simulink model "generic_uservehicle_truck"  (Simulink 10.3)
settings: Solver=ode45  StartTime=0.0  StopTime=inf  RelTol=1e-3  EnableMultiTasking=on
(part 1 of 4)
settings Model: Creator=fh  ModifiedByFormat=IPG  LastModifiedBy=IPG  MultithreadedSim=on  ExtModeAutoUpdateStatusClock=off
settings DataIOCC: LimitDataPoints=on  SignalLoggingName=sigsOut
settings OptimizationCC: BooleanDataType=off  InitFltsAndDblsToZero=on
settings DebuggingCC: SaveWithParameterizedLinksMsg=none  SignalResolutionControl=TryResolveAllWithWarning  MultiTaskDSMMsg=warning  MultiTaskCondExecSysMsg=none  SFExecutionAtInitializationDiag=warning
settings HardwareCC: TargetUnknown=on
settings CodeAppCC: MaxIdLength=63
settings GRTTargetCC: TargetFcnLib=ansi_tfl_tmw.mat

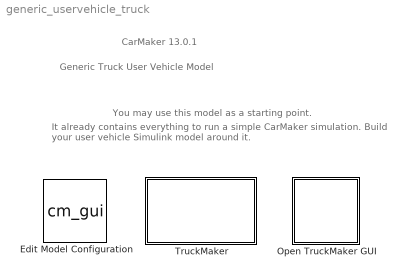
== system generic_uservehicle_truck ==
  note: Generic Truck User Vehicle Model
  note: CarMaker 13.0.1
  note: You may use this model as a starting point.
  note: It already contains everything to run a simple CarMaker simulation.
      | Build your user vehicle Simulink model around it.
  Edit Model Configuration : S-Function  FunctionName=cm_gui  SFunctionDeploymentMode=off  EnableBusSupport=off
      settings: OpenFcn=cmmodelconf('edit');
      mask Display: image(imread('ModelConfig.png'));
  Open TruckMaker GUI : Subsystem  LoadFcn=if ~length(which('cmself')), cmenv; end
      settings: OpenFcn=cmblockmagic('gui_fix_display'); TM_Simulink
      mask Display: image(imread('TruckMakerGUI.png'));
  TruckMaker : Subsystem  TreatAsAtomicUnit=on
      mask Display: image(imread('TruckMakerSys.png'));

== system generic_uservehicle_truck/Open TruckMaker GUI ==
  S-Function : S-Function  FunctionName=cm_gui  SFunctionDeploymentMode=off  EnableBusSupport=off

== system generic_uservehicle_truck/TruckMaker ==
  CM_FIRST : Subsystem
  CM_LAST : Subsystem
  DrivMan : Subsystem
  Ground : Ground
  Terminator : Terminator
  Vehicle : Subsystem
  VehicleControl : Subsystem
  wires:
  DrivMan/2(DrivMan.Out) -> VehicleControl/2(DrivMan.In)
  DrivMan/1(Sync_Out) -> VehicleControl/1(Sync_In)
  CM_FIRST/2(Env.Misc) -> DrivMan/2(Env.Misc)
  CM_FIRST/1(Sync_Out) -> DrivMan/1(Sync_In)
  CM_LAST/1(Sync_Out) -> Terminator/1
  Ground/1 -> CM_FIRST/1(Sync_In)
  Vehicle/1(Sync_Out) -> CM_LAST/1(Sync_In)
  VehicleControl/1(Sync_Out) -> Vehicle/1(Sync_In)
  VehicleControl/3(VhclCtrl.Steering) -> Vehicle/3(VhclCtrl.Steering)
  VehicleControl/4(Vhcl.Wheel.In) -> Vehicle/4(Vhcl.Wheel.In)
  VehicleControl/5(Vhcl.Misc) -> Vehicle/5(Vhcl.Misc)
  VehicleControl/6(VhclCtrl.Brake) -> Vehicle/6(VhclCtrl.Brake)
  VehicleControl/7(VhclCtrl.PT) -> Vehicle/7(VhclCtrl.PT)
  VehicleControl/2(Vhcl.Model.Source) -> Vehicle/2(Vhcl.Model.Source)

== system generic_uservehicle_truck/TruckMaker/CM_FIRST ==
  Sync_In : Inport
  BusCreator1 : BusCreator  Inputs=8
  BusCreator2 : BusCreator  Inputs=6
  Demux1 : Demux  Outputs=14
      settings: DisplayOption=none
  Environment : S-Function  FunctionName=TM_Sfun  Parameters='Environment'  SFunctionDeploymentMode=off  EnableBusSupport=off
  IoIn : S-Function  FunctionName=TM_Sfun  Parameters='IoIn'  SFunctionDeploymentMode=off  EnableBusSupport=off
  Terminator : Terminator
  Sync_Out : Outport  VectorParamsAs1DForOutWhenUnconnected=off
  Env.Misc : Outport  Port=2  VectorParamsAs1DForOutWhenUnconnected=off
  wires:
  BusCreator2/1 -> Terminator/1  "IF Environment (in)"
  BusCreator1/1 -> Env.Misc/1
  Demux1/14 -> BusCreator2/6  "Env sRoad"
  Demux1/13 -> BusCreator2/5  "Env PoI_GCS Elev"
  Demux1/12 -> BusCreator2/4  "Env PoI_GCS Lat"
  Demux1/11 -> BusCreator2/3  "Env PoI_GCS Long"
  Demux1/10 -> BusCreator2/2  "Env Time"
  Demux1/9 -> BusCreator2/1  "Env yDay"
  Demux1/8 -> BusCreator1/8  "Env WindVel_tot z"
  Demux1/7 -> BusCreator1/7  "Env WindVel_tot y"
  Demux1/6 -> BusCreator1/6  "Env WindVel_tot x"
  Demux1/5 -> BusCreator1/5  "Env SolarRadiation"
  Demux1/4 -> BusCreator1/4  "Env AirHumidity"
  Demux1/3 -> BusCreator1/3  "Env AirPressure"
  Demux1/2 -> BusCreator1/2  "Env AirDensity"
  Demux1/1 -> BusCreator1/1  "Env Temperature"
  Environment/2 -> Demux1/1
  Environment/1 -> Sync_Out/1
  IoIn/1 -> Environment/1
  Sync_In/1 -> IoIn/1

== system generic_uservehicle_truck/TruckMaker/CM_LAST ==
  Sync_In : Inport
  CM_User : S-Function  FunctionName=TM_Sfun  Parameters='CM_User'  SFunctionDeploymentMode=off  EnableBusSupport=off
  IoOut : S-Function  FunctionName=TM_Sfun  Parameters='IoOut'  SFunctionDeploymentMode=off  EnableBusSupport=off
  Sync_Out : Outport  VectorParamsAs1DForOutWhenUnconnected=off
  wires:
  IoOut/1 -> Sync_Out/1
  CM_User/1 -> IoOut/1
  Sync_In/1 -> CM_User/1

== system generic_uservehicle_truck/TruckMaker/DrivMan ==
  note: There's rarely a reason to override DrivMan signals.
      | Use the VehicleControl interface for this purpose.
  Sync_In : Inport
  Env.Misc : Inport  Port=2
  BusCreator : BusCreator  Inputs=20
  Demux : Demux  Outputs=20
      settings: DisplayOption=none
  DrivMan : S-Function  FunctionName=TM_Sfun  Parameters='DrivMan'  SFunctionDeploymentMode=off  EnableBusSupport=off
  Sync_Out : Outport  VectorParamsAs1DForOutWhenUnconnected=off
  DrivMan.Out : Outport  Port=2  VectorParamsAs1DForOutWhenUnconnected=off
  wires:
  Demux/8 -> BusCreator/8  "DrivMan SelectorCtrl"
  Demux/7 -> BusCreator/7  "DrivMan UserSignal4"
  Demux/6 -> BusCreator/6  "DrivMan UserSignal3"
  Demux/5 -> BusCreator/5  "DrivMan UserSignal2"
  Demux/4 -> BusCreator/4  "DrivMan UserSignal1"
  Demux/3 -> BusCreator/3  "DrivMan UserSignal0"
  Demux/2 -> BusCreator/2  "DrivMan Key"
  Demux/1 -> BusCreator/1  "DrivMan SST"
  Env.Misc/1 -> DrivMan/2
  Sync_In/1 -> DrivMan/1
  DrivMan/1 -> Sync_Out/1
  BusCreator/1 -> DrivMan.Out/1
  DrivMan/2 -> Demux/1
  Demux/9 -> BusCreator/9  "DrivMan DigitalSelectorCtrl0"
  Demux/10 -> BusCreator/10  "DrivMan DigitalSelectorCtrl1"
  Demux/11 -> BusCreator/11  "DrivMan DigitalSelectorCtrl2"
  Demux/20 -> BusCreator/20  "DrivMan Steering Trq"
  Demux/19 -> BusCreator/19  "DrivMan Steering AngAcc"
  Demux/18 -> BusCreator/18  "DrivMan Steering AngVel"
  Demux/17 -> BusCreator/17  "DrivMan Steering Ang"
  Demux/16 -> BusCreator/16  "DrivMan Gas"
  Demux/15 -> BusCreator/15  "DrivMan Clutch"
  Demux/14 -> BusCreator/14  "DrivMan BrakePark"
  Demux/13 -> BusCreator/13  "DrivMan Brake"
  Demux/12 -> BusCreator/12  "DrivMan GearNo"

== system generic_uservehicle_truck/TruckMaker/Vehicle ==
  note: The enabled subsystems allow for simultaneous availability of more than one vehicle.
      | Which one to use will be determined by the vehicle data set of the Test Run.
      | If this functionality is not needed, you may simplify your model by using
      | the relevant subsystem of the three as a drop-in replacement for the
      | 'Vehicle' subsystem you're currently looking at, as is done in most of the
      | CarMaker for Simulink example models.
      |
      | PLEASE NOTE: In CarMaker HIL-ds100x vehicle switching depending on
      | the vehicle data set is not available. To run the user vehicle, the command
      | line option -disablevehicle in the Model Configuration block is required.
  Sync_In : Inport
  Vhcl.Model.Source : Inport  Port=2
  VhclCtrl.Steering : Inport  Port=3
  Vhcl.Wheel.In : Inport  Port=4
  Vhcl.Misc : Inport  Port=5
  VhclCtrl.Brake : Inport  Port=6
  VhclCtrl.PT : Inport  Port=7
  IPG Vehicle : Subsystem
  Multiport Switch : MultiPortSwitch  InputSameDT=on
  User Vehicle (CM4SL) : Subsystem  TreatAsAtomicUnit=on
  User Vehicle (ModelMgr) : Subsystem  TreatAsAtomicUnit=on
  VehicleSource_BuiltIn : Subsystem  mask(Compare To Constant){relop===, const=1, OutDataTypeStr=boolean, ZeroCross=off}
      mask prompts: relop "Simulink:masks:Operator_MP"; const "Simulink:masks:ConstantValue_MP"; OutDataTypeStr "Simulink:masks:OutputDataType_MP"; ZeroCross "Simulink:masks:EnableZerocrossingDetection_MP"
      mask help: Simulink:masks:CompareToConstant_MD
      mask init:
      | blkName = gcb;
      | 
      | if strcmp(get_param(gcbh,'OutDataTypeStr'),'boolean')
      | 	setValue = 'boolean';
      | else
      | 	setValue = 'fixdt(0, 8)';
      | end
      | 
      | set_param([blkName,'/Compare'],'relop',relop, ...
      | 	'OutDataTypeStr', setValue, 'ZeroCross', ZeroCross);
      | 
      | str = [relop,' C']; %default
      | 
      | const_str = get_param(blkName, 'const');
      | 
      | if isempty(strfind(const_str, ' ')) && isempty(strfind(const_str, ','))
      |     % scalar or single expression
      |     if isempty(str2num(const_str))
      |         %expression
      |         str = [relop, ' ', const_str];
      |     elseif length(const) == 1
      |         str = [relop,' ',num2str(double(const))];
      |     end
      | end
      mask TypeOptions relop: == | ~= | < | <= | >= | >
      mask TypeOptions OutDataTypeStr: Simulink:masks:uint8 | Simulink:masks:boolean
      mask Callback ZeroCross: sl('zeroCrossEnable', gcbh);
      mask Display: disp(str)
  VehicleSource_CM4SL : Subsystem  mask(Compare To Constant){relop===, const=3, OutDataTypeStr=boolean, ZeroCross=off}
      mask prompts: relop "Simulink:masks:Operator_MP"; const "Simulink:masks:ConstantValue_MP"; OutDataTypeStr "Simulink:masks:OutputDataType_MP"; ZeroCross "Simulink:masks:EnableZerocrossingDetection_MP"
      mask help: Simulink:masks:CompareToConstant_MD
      mask init: same as generic_uservehicle_truck/TruckMaker/Vehicle/VehicleSource_BuiltIn
      mask TypeOptions relop: == | ~= | < | <= | >= | >
      mask TypeOptions OutDataTypeStr: Simulink:masks:uint8 | Simulink:masks:boolean
      mask Callback ZeroCross: sl('zeroCrossEnable', gcbh);
      mask Display: disp(str)
  VehicleSource_ModelMgr : Subsystem  mask(Compare To Constant){relop===, const=2, OutDataTypeStr=boolean, ZeroCross=off}
      mask prompts: relop "Simulink:masks:Operator_MP"; const "Simulink:masks:ConstantValue_MP"; OutDataTypeStr "Simulink:masks:OutputDataType_MP"; ZeroCross "Simulink:masks:EnableZerocrossingDetection_MP"
      mask help: Simulink:masks:CompareToConstant_MD
      mask init: same as generic_uservehicle_truck/TruckMaker/Vehicle/VehicleSource_BuiltIn
      mask TypeOptions relop: == | ~= | < | <= | >= | >
      mask TypeOptions OutDataTypeStr: Simulink:masks:uint8 | Simulink:masks:boolean
      mask Callback ZeroCross: sl('zeroCrossEnable', gcbh);
      mask Display: disp(str)
  Sync_Out : Outport  VectorParamsAs1DForOutWhenUnconnected=off
  wires:
  VhclCtrl.Steering/1 -> User Vehicle (CM4SL)/3(VhclCtrl.Steering), User Vehicle (ModelMgr)/3(VhclCtrl.Steering), IPG Vehicle/3(VhclCtrl.Steering)
  Vhcl.Wheel.In/1 -> User Vehicle (CM4SL)/4(Vhcl.Wheel.In), User Vehicle (ModelMgr)/4(Vhcl.Wheel.In), IPG Vehicle/4(Vhcl.Wheel.In)
  Vhcl.Misc/1 -> User Vehicle (CM4SL)/5(Vhcl.Misc), User Vehicle (ModelMgr)/5(Vhcl.Misc), IPG Vehicle/5(Vhcl.Misc)
  VehicleSource_BuiltIn/1(y) -> IPG Vehicle/Enable
  VhclCtrl.Brake/1 -> User Vehicle (CM4SL)/6(VhclCtrl.Brake), User Vehicle (ModelMgr)/6(VhclCtrl.Brake), IPG Vehicle/6(VhclCtrl.Brake)
  VhclCtrl.PT/1 -> User Vehicle (CM4SL)/7(VhclCtrl.PT), User Vehicle (ModelMgr)/7(VhclCtrl.PT), IPG Vehicle/7(VhclCtrl.PT)
  Sync_In/1 -> User Vehicle (CM4SL)/1(Sync_In), User Vehicle (ModelMgr)/1(Sync_In), IPG Vehicle/1(Sync_In)
  Vhcl.Model.Source/1 -> User Vehicle (CM4SL)/2(Vhcl.Model.Source), VehicleSource_ModelMgr/1(u), VehicleSource_BuiltIn/1(u), Multiport Switch/1, IPG Vehicle/2(Vhcl.Model.Source), User Vehicle (ModelMgr)/2(Vhcl.Model.Source), VehicleSource_CM4SL/1(u)
  VehicleSource_CM4SL/1(y) -> User Vehicle (CM4SL)/Enable
  VehicleSource_ModelMgr/1(y) -> User Vehicle (ModelMgr)/Enable
  IPG Vehicle/1(Sync_Out) -> Multiport Switch/2
  User Vehicle (ModelMgr)/1(Sync_Out) -> Multiport Switch/3
  User Vehicle (CM4SL)/1(Sync_Out) -> Multiport Switch/4
  Multiport Switch/1 -> Sync_Out/1

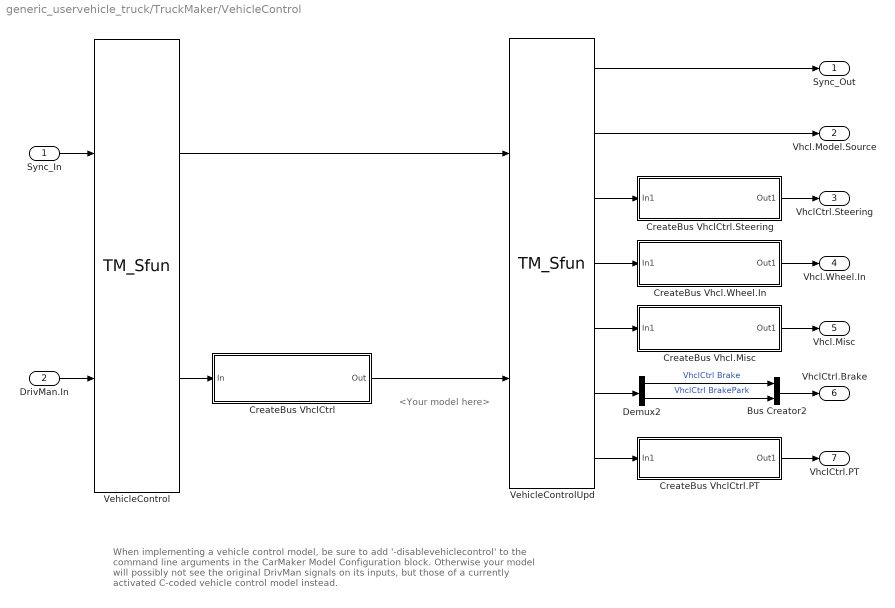
== system generic_uservehicle_truck/TruckMaker/VehicleControl ==
  note: <Your model here>
  note: When implementing a vehicle control model,
      | be sure to add '-disablevehiclecontrol' to the command line arguments
      | in the CarMaker Model Configuration block.
      | Otherwise your model will possibly not see the original DrivMan signals
      | on its inputs, but those of a currently activated C-coded vehicle control model instead.
  Sync_In : Inport
  DrivMan.In : Inport  Port=2
  Bus Creator2 : BusCreator  Inputs=2
  CreateBus Vhcl.Misc : Subsystem
  CreateBus Vhcl.Wheel.In : Subsystem
  CreateBus VhclCtrl : Subsystem
  CreateBus VhclCtrl.PT : Subsystem
  CreateBus VhclCtrl.Steering : Subsystem
  Demux2 : Demux  Outputs=2
      settings: DisplayOption=none
  VehicleControl : S-Function  FunctionName=TM_Sfun  Parameters='VehicleControl'  SFunctionDeploymentMode=off  EnableBusSupport=off
  VehicleControlUpd : S-Function  FunctionName=TM_Sfun  Parameters='VehicleControlUpd'  SFunctionDeploymentMode=off  EnableBusSupport=off
  Sync_Out : Outport  VectorParamsAs1DForOutWhenUnconnected=off
  Vhcl.Model.Source : Outport  Port=2  VectorParamsAs1DForOutWhenUnconnected=off
  VhclCtrl.Steering : Outport  Port=3  VectorParamsAs1DForOutWhenUnconnected=off
  Vhcl.Wheel.In : Outport  Port=4  VectorParamsAs1DForOutWhenUnconnected=off
  Vhcl.Misc : Outport  Port=5  VectorParamsAs1DForOutWhenUnconnected=off
  VhclCtrl.Brake : Outport  Port=6  VectorParamsAs1DForOutWhenUnconnected=off
  VhclCtrl.PT : Outport  Port=7  VectorParamsAs1DForOutWhenUnconnected=off
  wires:
  VehicleControlUpd/2 -> Vhcl.Model.Source/1
  VehicleControlUpd/4 -> CreateBus Vhcl.Wheel.In/1(In1)
  VehicleControlUpd/5 -> CreateBus Vhcl.Misc/1(In1)
  VehicleControlUpd/6 -> Demux2/1
  VehicleControlUpd/7 -> CreateBus VhclCtrl.PT/1(In1)
  VehicleControlUpd/3 -> CreateBus VhclCtrl.Steering/1(In1)
  CreateBus Vhcl.Misc/1(Out1) -> Vhcl.Misc/1
  CreateBus Vhcl.Wheel.In/1(Out1) -> Vhcl.Wheel.In/1
  DrivMan.In/1 -> VehicleControl/2
  CreateBus VhclCtrl/1(Out) -> VehicleControlUpd/2
  VehicleControl/1 -> VehicleControlUpd/1
  VehicleControl/2 -> CreateBus VhclCtrl/1(In)
  Sync_In/1 -> VehicleControl/1
  CreateBus VhclCtrl.PT/1(Out1) -> VhclCtrl.PT/1
  Bus Creator2/1 -> VhclCtrl.Brake/1
  CreateBus VhclCtrl.Steering/1(Out1) -> VhclCtrl.Steering/1
  VehicleControlUpd/1 -> Sync_Out/1
  Demux2/2 -> Bus Creator2/2  "VhclCtrl BrakePark"
  Demux2/1 -> Bus Creator2/1  "VhclCtrl Brake"

== system generic_uservehicle_truck/TruckMaker/Vehicle/IPG Vehicle ==
  Sync_In : Inport
  Vhcl.Model.Source : Inport  Port=2
  VhclCtrl.Steering : Inport  Port=3
  Vhcl.Wheel.In : Inport  Port=4
  Vhcl.Misc : Inport  Port=5
  VhclCtrl.Brake : Inport  Port=6
  VhclCtrl.PT : Inport  Port=7
  Enable : EnablePort
  Brake : Subsystem
  CarAndTrailer : Subsystem
  PowerTrain : Subsystem
  Stop Simulation : Stop
  VehicleSource_BuiltIn : Subsystem  mask(Compare To Constant){relop=~=, const=1, OutDataTypeStr=boolean, ZeroCross=off}
      mask prompts: relop "Simulink:masks:Operator_MP"; const "Simulink:masks:ConstantValue_MP"; OutDataTypeStr "Simulink:masks:OutputDataType_MP"; ZeroCross "Simulink:masks:EnableZerocrossingDetection_MP"
      mask help: Simulink:masks:CompareToConstant_MD
      mask init: same as generic_uservehicle_truck/TruckMaker/Vehicle/VehicleSource_BuiltIn
      mask TypeOptions relop: == | ~= | < | <= | >= | >
      mask TypeOptions OutDataTypeStr: Simulink:masks:uint8 | Simulink:masks:boolean
      mask Callback ZeroCross: sl('zeroCrossEnable', gcbh);
      mask Display: disp(str)
  Sync_Out : Outport  VectorParamsAs1DForOutWhenUnconnected=off
  wires:
  VhclCtrl.PT/1 -> PowerTrain/3(VhclCtrl.PT)
  Brake/1(Sync_Out) -> PowerTrain/1(Sync_In)
  CarAndTrailer/1(Sync_Out) -> Brake/1(Sync_In)
  CarAndTrailer/2(Brake.IF.In) -> Brake/2(Brake.IF.In)
  VhclCtrl.Brake/1 -> Brake/3(VhclCtrl.Brake)
  PowerTrain/1(Sync_Out) -> Sync_Out/1
  Vhcl.Misc/1 -> CarAndTrailer/4(Vhcl.Misc)
  Vhcl.Wheel.In/1 -> CarAndTrailer/3(Vhcl.Wheel.In)
  VhclCtrl.Steering/1 -> CarAndTrailer/2(VhclCtrl.Steering)
  Sync_In/1 -> CarAndTrailer/1(Sync_In)
  Vhcl.Model.Source/1 -> VehicleSource_BuiltIn/1(u)
  VehicleSource_BuiltIn/1(y) -> Stop Simulation/1
  Brake/2(Vhcl.Wheel.PT) -> PowerTrain/2(Vhcl.Wheel.PT)

== system generic_uservehicle_truck/TruckMaker/Vehicle/User Vehicle (CM4SL) ==
  Sync_In : Inport
  Vhcl.Model.Source : Inport  Port=2
  VhclCtrl.Steering : Inport  Port=3
  Vhcl.Wheel.In : Inport  Port=4
  Vhcl.Misc : Inport  Port=5
  VhclCtrl.Brake : Inport  Port=6
  VhclCtrl.PT : Inport  Port=7
  Enable : EnablePort
  Brake : Subsystem
  CarAndTrailer : Subsystem
  PowerTrain : Subsystem
  Stop Simulation : Stop
  VehicleSource_CM4SL : Subsystem  mask(Compare To Constant){relop=~=, const=3, OutDataTypeStr=boolean, ZeroCross=off}
      mask prompts: relop "Simulink:masks:Operator_MP"; const "Simulink:masks:ConstantValue_MP"; OutDataTypeStr "Simulink:masks:OutputDataType_MP"; ZeroCross "Simulink:masks:EnableZerocrossingDetection_MP"
      mask help: Simulink:masks:CompareToConstant_MD
      mask init: same as generic_uservehicle_truck/TruckMaker/Vehicle/VehicleSource_BuiltIn
      mask TypeOptions relop: == | ~= | < | <= | >= | >
      mask TypeOptions OutDataTypeStr: Simulink:masks:uint8 | Simulink:masks:boolean
      mask Callback ZeroCross: sl('zeroCrossEnable', gcbh);
      mask Display: disp(str)
  Sync_Out : Outport  VectorParamsAs1DForOutWhenUnconnected=off
  wires:
  Brake/2(Vhcl.Wheel.PT) -> PowerTrain/2(Vhcl.Wheel.PT)
  Brake/1(Sync_Out) -> PowerTrain/1(Sync_In)
  Sync_In/1 -> CarAndTrailer/1(Sync_In)
  VhclCtrl.Steering/1 -> CarAndTrailer/2(VhclCtrl.Steering)
  Vhcl.Wheel.In/1 -> CarAndTrailer/3(Vhcl.Wheel.In)
  Vhcl.Misc/1 -> CarAndTrailer/4(Vhcl.Misc)
  PowerTrain/1(Sync_Out) -> Sync_Out/1
  VhclCtrl.Brake/1 -> Brake/3(VhclCtrl.Brake)
  CarAndTrailer/2(Brake.IF.In) -> Brake/2(Brake.IF.In)
  CarAndTrailer/1(Sync_Out) -> Brake/1(Sync_In)
  VhclCtrl.PT/1 -> PowerTrain/3(VhclCtrl.PT)
  Vhcl.Model.Source/1 -> VehicleSource_CM4SL/1(u)
  VehicleSource_CM4SL/1(y) -> Stop Simulation/1

== system generic_uservehicle_truck/TruckMaker/Vehicle/User Vehicle (ModelMgr) ==
  Sync_In : Inport
  Vhcl.Model.Source : Inport  Port=2
  VhclCtrl.Steering : Inport  Port=3
  Vhcl.Wheel.In : Inport  Port=4
  Vhcl.Misc : Inport  Port=5
  VhclCtrl.Brake : Inport  Port=6
  VhclCtrl.PT : Inport  Port=7
  Enable : EnablePort
  Brake : Subsystem
  CarAndTrailer : Subsystem
  PowerTrain : Subsystem
  Stop Simulation : Stop
  VehicleSource_ModelMgr : Subsystem  mask(Compare To Constant){relop=~=, const=2, OutDataTypeStr=boolean, ZeroCross=off}
      mask prompts: relop "Simulink:masks:Operator_MP"; const "Simulink:masks:ConstantValue_MP"; OutDataTypeStr "Simulink:masks:OutputDataType_MP"; ZeroCross "Simulink:masks:EnableZerocrossingDetection_MP"
      mask help: Simulink:masks:CompareToConstant_MD
      mask init: same as generic_uservehicle_truck/TruckMaker/Vehicle/VehicleSource_BuiltIn
      mask TypeOptions relop: == | ~= | < | <= | >= | >
      mask TypeOptions OutDataTypeStr: Simulink:masks:uint8 | Simulink:masks:boolean
      mask Callback ZeroCross: sl('zeroCrossEnable', gcbh);
      mask Display: disp(str)
  Sync_Out : Outport  VectorParamsAs1DForOutWhenUnconnected=off
  wires:
  Brake/1(Sync_Out) -> PowerTrain/1(Sync_In)
  Brake/2(Vhcl.Wheel.PT) -> PowerTrain/2(Vhcl.Wheel.PT)
  Vhcl.Model.Source/1 -> VehicleSource_ModelMgr/1(u)
  Sync_In/1 -> CarAndTrailer/1(Sync_In)
  VhclCtrl.Brake/1 -> Brake/3(VhclCtrl.Brake)
  VhclCtrl.PT/1 -> PowerTrain/3(VhclCtrl.PT)
  PowerTrain/1(Sync_Out) -> Sync_Out/1
  CarAndTrailer/1(Sync_Out) -> Brake/1(Sync_In)
  CarAndTrailer/2(Brake.IF.In) -> Brake/2(Brake.IF.In)
  Vhcl.Misc/1 -> CarAndTrailer/4(Vhcl.Misc)
  Vhcl.Wheel.In/1 -> CarAndTrailer/3(Vhcl.Wheel.In)
  VhclCtrl.Steering/1 -> CarAndTrailer/2(VhclCtrl.Steering)
  VehicleSource_ModelMgr/1(y) -> Stop Simulation/1

== system generic_uservehicle_truck/TruckMaker/Vehicle/VehicleSource_BuiltIn ==
  u : Inport
  Compare : RelationalOperator  Operator===  OutDataTypeStr=boolean  ZeroCross=off  RndMeth=Nearest  InputSameDT=on
  Constant : Constant  DisableCoverage=on  Value=const  OutDataTypeStr=Inherit: Inherit via back propagation
  y : Outport  VectorParamsAs1DForOutWhenUnconnected=off
  wires:
  u/1 -> Compare/1
  Constant/1 -> Compare/2
  Compare/1 -> y/1

== system generic_uservehicle_truck/TruckMaker/Vehicle/VehicleSource_CM4SL ==
  u : Inport
  Compare : RelationalOperator  Operator===  OutDataTypeStr=boolean  ZeroCross=off  RndMeth=Nearest  InputSameDT=on
  Constant : Constant  DisableCoverage=on  Value=const  OutDataTypeStr=Inherit: Inherit via back propagation
  y : Outport  VectorParamsAs1DForOutWhenUnconnected=off
  wires:
  u/1 -> Compare/1
  Constant/1 -> Compare/2
  Compare/1 -> y/1

== system generic_uservehicle_truck/TruckMaker/Vehicle/VehicleSource_ModelMgr ==
  u : Inport
  Compare : RelationalOperator  Operator===  OutDataTypeStr=boolean  ZeroCross=off  RndMeth=Nearest  InputSameDT=on
  Constant : Constant  DisableCoverage=on  Value=const  OutDataTypeStr=Inherit: Inherit via back propagation
  y : Outport  VectorParamsAs1DForOutWhenUnconnected=off
  wires:
  u/1 -> Compare/1
  Constant/1 -> Compare/2
  Compare/1 -> y/1

== system generic_uservehicle_truck/TruckMaker/VehicleControl/CreateBus Vhcl.Misc ==
  In1 : Inport
  Bus Creator5 : BusCreator  Inputs=11
  Demux5 : Demux  Outputs=11
      settings: DisplayOption=none
  Out1 : Outport  VectorParamsAs1DForOutWhenUnconnected=off
  wires:
  Demux5/11 -> Bus Creator5/11  "Vhcl Wind_vel_0 z"
  Demux5/10 -> Bus Creator5/10  "Vhcl Wind_vel_0 y"
  Demux5/9 -> Bus Creator5/9  "Vhcl Wind_vel_0 x"
  Demux5/8 -> Bus Creator5/8  "Vhcl DL2BdyEng y"
  Demux5/7 -> Bus Creator5/7  "Vhcl DL2BdyEng x"
  Demux5/6 -> Bus Creator5/6  "Vhcl TrqDL2Bdy1B z"
  Demux5/5 -> Bus Creator5/5  "Vhcl TrqDL2Bdy1B y"
  Demux5/4 -> Bus Creator5/4  "Vhcl TrqDL2Bdy1B x"
  Demux5/3 -> Bus Creator5/3  "Vhcl Trq_DL2Bdy1 z"
  In1/1 -> Demux5/1
  Bus Creator5/1 -> Out1/1
  Demux5/2 -> Bus Creator5/2  "Vhcl Trq_DL2Bdy1 y"
  Demux5/1 -> Bus Creator5/1  "Vhcl Trq_DL2Bdy1 x"

== system generic_uservehicle_truck/TruckMaker/VehicleControl/CreateBus Vhcl.Wheel.In ==
  In1 : Inport
  Bus Creator1 : BusCreator  Inputs=36
  Demux1 : Demux  Outputs=36
      settings: DisplayOption=none
  Out1 : Outport  VectorParamsAs1DForOutWhenUnconnected=off
  wires:
  Demux1/36 -> Bus Creator1/36  "Vhcl Wheel RR4 rotv"
  Demux1/35 -> Bus Creator1/35  "Vhcl Wheel RR4 Trq_DL2WC"
  Demux1/34 -> Bus Creator1/34  "Vhcl Wheel RR4 Trq_B2WC"
  Demux1/33 -> Bus Creator1/33  "Vhcl Wheel RL4 rotv"
  Demux1/32 -> Bus Creator1/32  "Vhcl Wheel RL4 Trq_DL2WC"
  Demux1/31 -> Bus Creator1/31  "Vhcl Wheel RL4 Trq_B2WC"
  Demux1/30 -> Bus Creator1/30  "Vhcl Wheel RR3 rotv"
  Demux1/29 -> Bus Creator1/29  "Vhcl Wheel RR3 Trq_DL2WC"
  Demux1/28 -> Bus Creator1/28  "Vhcl Wheel RR3 Trq_B2WC"
  Demux1/27 -> Bus Creator1/27  "Vhcl Wheel RL3 rotv"
  Demux1/26 -> Bus Creator1/26  "Vhcl Wheel RL3 Trq_DL2WC"
  Demux1/25 -> Bus Creator1/25  "Vhcl Wheel RL3 Trq_B2WC"
  Demux1/12 -> Bus Creator1/12  "Vhcl Wheel RR rotv"
  Demux1/11 -> Bus Creator1/11  "Vhcl Wheel RR Trq_DL2WC"
  Demux1/10 -> Bus Creator1/10  "Vhcl Wheel RR Trq_B2WC"
  Demux1/9 -> Bus Creator1/9  "Vhcl Wheel RL rotv"
  Demux1/8 -> Bus Creator1/8  "Vhcl Wheel RL Trq_DL2WC"
  Demux1/7 -> Bus Creator1/7  "Vhcl Wheel RL Trq_B2WC"
  Demux1/6 -> Bus Creator1/6  "Vhcl Wheel FR rotv"
  Demux1/5 -> Bus Creator1/5  "Vhcl Wheel FR Trq_DL2WC"
  Demux1/4 -> Bus Creator1/4  "Vhcl Wheel FR Trq_B2WC"
  Demux1/3 -> Bus Creator1/3  "Vhcl Wheel FL rotv"
  Demux1/2 -> Bus Creator1/2  "Vhcl Wheel FL Trq_DL2WC"
  Demux1/1 -> Bus Creator1/1  "Vhcl Wheel FL Trq_B2WC"
  Bus Creator1/1 -> Out1/1
  In1/1 -> Demux1/1
  Demux1/24 -> Bus Creator1/24  "Vhcl Wheel FR2 rotv"
  Demux1/23 -> Bus Creator1/23  "Vhcl Wheel FR2 Trq_DL2WC"
  Demux1/22 -> Bus Creator1/22  "Vhcl Wheel FR2 Trq_B2WC"
  Demux1/21 -> Bus Creator1/21  "Vhcl Wheel FL2 rotv"
  Demux1/20 -> Bus Creator1/20  "Vhcl Wheel FL2 Trq_DL2WC"
  Demux1/19 -> Bus Creator1/19  "Vhcl Wheel FL2 Trq_B2WC"
  Demux1/18 -> Bus Creator1/18  "Vhcl Wheel RR2 rotv"
  Demux1/17 -> Bus Creator1/17  "Vhcl Wheel RR2 Trq_DL2WC"
  Demux1/16 -> Bus Creator1/16  "Vhcl Wheel RR2 Trq_B2WC"
  Demux1/15 -> Bus Creator1/15  "Vhcl Wheel RL2 rotv"
  Demux1/14 -> Bus Creator1/14  "Vhcl Wheel RL2 Trq_DL2WC"
  Demux1/13 -> Bus Creator1/13  "Vhcl Wheel RL2 Trq_B2WC"

== system generic_uservehicle_truck/TruckMaker/VehicleControl/CreateBus VhclCtrl ==
  In : Inport
  BusCreator : BusCreator  Inputs=29
  Demux : Demux  Outputs=29
      settings: DisplayOption=none
  Out : Outport  VectorParamsAs1DForOutWhenUnconnected=off
  wires:
  Demux/29 -> BusCreator/29  "VhclCtrl Lights Reverse"
  Demux/28 -> BusCreator/28  "VhclCtrl Lights Brake"
  Demux/27 -> BusCreator/27  "VhclCtrl Lights FogRear"
  Demux/26 -> BusCreator/26  "VhclCtrl Lights FogFrontR"
  Demux/25 -> BusCreator/25  "VhclCtrl Lights FogFrontL"
  Demux/24 -> BusCreator/24  "VhclCtrl Lights IndR"
  Demux/23 -> BusCreator/23  "VhclCtrl Lights IndL"
  Demux/22 -> BusCreator/22  "VhclCtrl Lights ParkR"
  Demux/21 -> BusCreator/21  "VhclCtrl Lights ParkL"
  Demux/20 -> BusCreator/20  "VhclCtrl Lights Daytime"
  Demux/19 -> BusCreator/19  "VhclCtrl Lights HighBeam"
  Demux/18 -> BusCreator/18  "VhclCtrl Lights LowBeam"
  Demux/17 -> BusCreator/17  "VhclCtrl Steering Trq"
  Demux/16 -> BusCreator/16  "VhclCtrl Steering AngAcc"
  Demux/15 -> BusCreator/15  "VhclCtrl Steering AngVel"
  Demux/14 -> BusCreator/14  "VhclCtrl Steering Ang"
  Demux/13 -> BusCreator/13  "VhclCtrl Gas"
  Demux/12 -> BusCreator/12  "VhclCtrl Clutch"
  Demux/11 -> BusCreator/11  "VhclCtrl BrakePark"
  Demux/10 -> BusCreator/10  "VhclCtrl Brake"
  Demux/9 -> BusCreator/9  "VhclCtrl SelectorCtrl"
  Demux/8 -> BusCreator/8  "VhclCtrl GearNo"
  Demux/7 -> BusCreator/7  "VhclCtrl UserSignal4"
  Demux/6 -> BusCreator/6  "VhclCtrl UserSignal3"
  Demux/5 -> BusCreator/5  "VhclCtrl UserSignal2"
  Demux/4 -> BusCreator/4  "VhclCtrl UserSignal1"
  Demux/3 -> BusCreator/3  "VhclCtrl UserSignal0"
  Demux/2 -> BusCreator/2  "VhclCtrl Key"
  Demux/1 -> BusCreator/1  "VhclCtrl SST"
  BusCreator/1 -> Out/1
  In/1 -> Demux/1

== system generic_uservehicle_truck/TruckMaker/VehicleControl/CreateBus VhclCtrl.PT ==
  In1 : Inport
  BusCreator1 : BusCreator  Inputs=12
  Demux1 : Demux  Outputs=12
      settings: DisplayOption=none
  Out1 : Outport  VectorParamsAs1DForOutWhenUnconnected=off
  wires:
  Demux1/12 -> BusCreator1/12  "VhclCtrl Brake"
  Demux1/11 -> BusCreator1/11  "VhclCtrl Gas"
  Demux1/10 -> BusCreator1/10  "VhclCtrl Clutch"
  Demux1/9 -> BusCreator1/9  "VhclCtrl SelectorCtrl"
  Demux1/8 -> BusCreator1/8  "VhclCtrl GearNo"
  Demux1/7 -> BusCreator1/7  "VhclCtrl UserSignal4"
  Demux1/6 -> BusCreator1/6  "VhclCtrl UserSignal3"
  Demux1/5 -> BusCreator1/5  "VhclCtrl UserSignal2"
  Demux1/4 -> BusCreator1/4  "VhclCtrl UserSignal1"
  Demux1/3 -> BusCreator1/3  "VhclCtrl UserSignal0"
  Demux1/2 -> BusCreator1/2  "VhclCtrl Key"
  Demux1/1 -> BusCreator1/1  "VhclCtrl SST"
  In1/1 -> Demux1/1
  BusCreator1/1 -> Out1/1

== system generic_uservehicle_truck/TruckMaker/VehicleControl/CreateBus VhclCtrl.Steering ==
  In1 : Inport
  Bus Creator : BusCreator  Inputs=5
  Demux : Demux  Outputs=5
      settings: DisplayOption=none
  Out1 : Outport  VectorParamsAs1DForOutWhenUnconnected=off
  wires:
  In1/1 -> Demux/1
  Bus Creator/1 -> Out1/1
  Demux/1 -> Bus Creator/1  "VhclCtrl Steering Ang"
  Demux/5 -> Bus Creator/5  "VhclCtrl Steering ByTrq"
  Demux/3 -> Bus Creator/3  "VhclCtrl Steering AngAcc"
  Demux/2 -> Bus Creator/2  "VhclCtrl Steering AngVel"
  Demux/4 -> Bus Creator/4  "VhclCtrl Steering Trq"

== system generic_uservehicle_truck/TruckMaker/Vehicle/IPG Vehicle/Brake ==
  note: <Your model here>
  note: When replacing the entire braking system,
      | be sure to disable the IPG brake model by using the brake
      | model 'Model Manager off' in the vehicle GUI.
  Sync_In : Inport
  Brake.IF.In : Inport  Port=2
  VhclCtrl.Brake : Inport  Port=3
  Brake : S-Function  FunctionName=TM_Sfun  Parameters='Brake'  SFunctionDeploymentMode=off  EnableBusSupport=off
  BrakeUpd : S-Function  FunctionName=TM_Sfun  Parameters='BrakeUpd'  SFunctionDeploymentMode=off  EnableBusSupport=off
  BusCreator : BusCreator  Inputs=48
  CreateBus Vhcl.Wheel.PT : Subsystem
  Demux : Demux  Outputs=48
      settings: DisplayOption=none
  Sync_Out : Outport  VectorParamsAs1DForOutWhenUnconnected=off
  Vhcl.Wheel.PT : Outport  Port=2  VectorParamsAs1DForOutWhenUnconnected=off
  wires:
  Demux/1 -> BusCreator/1  "Brake IF Trq_WB FL"
  Demux/2 -> BusCreator/2  "Brake IF Trq_WB FR"
  Demux/3 -> BusCreator/3  "Brake IF Trq_WB RL"
  Demux/4 -> BusCreator/4  "Brake IF Trq_WB RR"
  Demux/5 -> BusCreator/5  "Brake IF Trq_WB RL2"
  Demux/6 -> BusCreator/6  "Brake IF Trq_WB RR2"
  Demux/7 -> BusCreator/7  "Brake IF Trq_WB FL2"
  Demux/8 -> BusCreator/8  "Brake IF Trq_WB FR2"
  Demux/9 -> BusCreator/9  "Brake IF Trq_WB RL3"
  Demux/10 -> BusCreator/10  "Brake IF Trq_WB RR3"
  Demux/11 -> BusCreator/11  "Brake IF Trq_WB RL4"
  Demux/12 -> BusCreator/12  "Brake IF Trq_WB RR4"
  Demux/13 -> BusCreator/13  "Brake IF Trq_PB FL"
  Demux/14 -> BusCreator/14  "Brake IF Trq_PB FR"
  Demux/15 -> BusCreator/15  "Brake IF Trq_PB RL"
  Demux/16 -> BusCreator/16  "Brake IF Trq_PB RR"
  Demux/17 -> BusCreator/17  "Brake IF Trq_PB RL2"
  Demux/18 -> BusCreator/18  "Brake IF Trq_PB RR2"
  Demux/19 -> BusCreator/19  "Brake IF Trq_PB FL2"
  Demux/20 -> BusCreator/20  "Brake IF Trq_PB FR2"
  Demux/21 -> BusCreator/21  "Brake IF Trq_PB RL3"
  Demux/22 -> BusCreator/22  "Brake IF Trq_PB RR3"
  Demux/23 -> BusCreator/23  "Brake IF Trq_PB RL4"
  Demux/24 -> BusCreator/24  "Brake IF Trq_PB RR4"
  Demux/25 -> BusCreator/25  "Brake IF Trq_Reg_trg FL"
  Demux/26 -> BusCreator/26  "Brake IF Trq_Reg_trg FR"
  Demux/27 -> BusCreator/27  "Brake IF Trq_Reg_trg RL"
  Demux/28 -> BusCreator/28  "Brake IF Trq_Reg_trg RR"
  Demux/29 -> BusCreator/29  "Brake IF Trq_Reg_trg RL2"
  Demux/30 -> BusCreator/30  "Brake IF Trq_Reg_trg RR2"
  Demux/31 -> BusCreator/31  "Brake IF Trq_Reg_trg FL2"
  Demux/32 -> BusCreator/32  "Brake IF Trq_Reg_trg FR2"
  Demux/33 -> BusCreator/33  "Brake IF Trq_Reg_trg RL3"
  Demux/34 -> BusCreator/34  "Brake IF Trq_Reg_trg RR3"
  Demux/35 -> BusCreator/35  "Brake IF Trq_Reg_trg RL4"
  Demux/36 -> BusCreator/36  "Brake IF Trq_Reg_trg RR4"
  Demux/37 -> BusCreator/37  "Brake IF Trq_DriveSrc_trg d0"
  Demux/38 -> BusCreator/38  "Brake IF Trq_DriveSrc_trg d1"
  Demux/39 -> BusCreator/39  "Brake IF Trq_DriveSrc_trg d2"
  Demux/40 -> BusCreator/40  "Brake IF Trq_DriveSrc_trg d3"
  Demux/41 -> BusCreator/41  "Brake IF Trq_DriveSrc_trg d4"
  Demux/42 -> BusCreator/42  "Brake IF Trq_DriveSrc_trg d5"
  Demux/43 -> BusCreator/43  "Brake IF Trq_DriveSrc_trg d6"
  Demux/44 -> BusCreator/44  "Brake IF Trq_DriveSrc_trg d7"
  Demux/45 -> BusCreator/45  "Brake IF Trq_DriveSrc_trg d8"
  Demux/46 -> BusCreator/46  "Brake IF Trq_DriveSrc_trg d9"
  Demux/47 -> BusCreator/47  "Brake IF Trq_DriveSrc_trg d10"
  Demux/48 -> BusCreator/48  "Brake IF Trq_DriveSrc_trg d11"
  BusCreator/1 -> BrakeUpd/2
  Brake/2 -> Demux/1
  BrakeUpd/1 -> Sync_Out/1
  Brake/1 -> BrakeUpd/1  "Sync"
  Brake.IF.In/1 -> Brake/2
  VhclCtrl.Brake/1 -> Brake/3
  Sync_In/1 -> Brake/1
  BrakeUpd/2 -> CreateBus Vhcl.Wheel.PT/1(In)
  CreateBus Vhcl.Wheel.PT/1(Out) -> Vhcl.Wheel.PT/1

== system generic_uservehicle_truck/TruckMaker/Vehicle/IPG Vehicle/CarAndTrailer ==
  Sync_In : Inport
  VhclCtrl.Steering : Inport  Port=2
  Vhcl.Wheel.In : Inport  Port=3
  Vhcl.Misc : Inport  Port=4
  CarAndTrailerUpd : Subsystem
  Forces : Subsystem
  Ground : Ground
  Kinematics : Subsystem
  Kinetics : Subsystem
  Steering : Subsystem
  Terminator : Terminator
  Terminator1 : Terminator
  Trailer : Subsystem
  Sync_Out : Outport  VectorParamsAs1DForOutWhenUnconnected=off
  Brake.IF.In : Outport  Port=2  VectorParamsAs1DForOutWhenUnconnected=off
  wires:
  Trailer/16(Vhcl.Wheel.RR4) -> CarAndTrailerUpd/16(Vhcl.Wheel.RR4)
  Trailer/15(Vhcl.Wheel.RL4) -> CarAndTrailerUpd/15(Vhcl.Wheel.RL4)
  Trailer/14(Vhcl.Wheel.RR3) -> CarAndTrailerUpd/14(Vhcl.Wheel.RR3)
  Trailer/13(Vhcl.Wheel.RL3) -> CarAndTrailerUpd/13(Vhcl.Wheel.RL3)
  Ground/1 -> CarAndTrailerUpd/18(Vhcl.Fr1A)
  Trailer/17(Car.Hitch.FrcTrq) -> CarAndTrailerUpd/17(Car.Hitch.FrcTrq)
  Trailer/12(Vhcl.Wheel.FR2) -> CarAndTrailerUpd/12(Vhcl.Wheel.FR2)
  Trailer/11(Vhcl.Wheel.FL2) -> CarAndTrailerUpd/11(Vhcl.Wheel.FL2)
  Trailer/10(Vhcl.Wheel.RR2) -> CarAndTrailerUpd/10(Vhcl.Wheel.RR2)
  Trailer/9(Vhcl.Wheel.RL2) -> CarAndTrailerUpd/9(Vhcl.Wheel.RL2)
  Trailer/8(Vhcl.Wheel.RR) -> CarAndTrailerUpd/8(Vhcl.Wheel.RR)
  Trailer/7(Vhcl.Wheel.RL) -> CarAndTrailerUpd/7(Vhcl.Wheel.RL)
  Trailer/6(Vhcl.Wheel.FR) -> CarAndTrailerUpd/6(Vhcl.Wheel.FR)
  Trailer/5(Vhcl.Wheel.FL) -> CarAndTrailerUpd/5(Vhcl.Wheel.FL)
  Trailer/4(Vhcl.PoI) -> CarAndTrailerUpd/4(Vhcl.PoI)
  Trailer/3(Vhcl.Motion) -> CarAndTrailerUpd/3(Vhcl.Motion)
  Trailer/2(Vhcl.Steering) -> CarAndTrailerUpd/2(Vhcl.Steering)
  Trailer/1(Sync_Out) -> CarAndTrailerUpd/1(Sync_In)
  CarAndTrailerUpd/2(Brake.IF.In) -> Brake.IF.In/1
  CarAndTrailerUpd/1(Sync_Out) -> Sync_Out/1
  Vhcl.Misc/1 -> Terminator1/1
  Vhcl.Wheel.In/1 -> Terminator/1
  Kinetics/6(WheelCarrier.Misc) -> Trailer/6(WheelCarrier.Misc)
  Kinetics/5(Car.Trq_T2W) -> Trailer/5(Car.Trq_T2W)
  Steering/2(Steer.IF) -> Kinematics/2(Steer.IF)
  Kinetics/4(Car.Fr1) -> Trailer/4(Car.Fr1)
  Kinetics/3(Car.Hitch) -> Trailer/3(Car.Hitch)
  Kinetics/2(Trailer.Load) -> Trailer/2(Trailer.Load)
  VhclCtrl.Steering/1 -> Steering/2(VhclCtrl.Steering)
  Sync_In/1 -> Steering/1(Sync_In)
  Steering/1(Sync_Out) -> Kinematics/1(Sync_In)
  Kinetics/1(Sync_Out) -> Trailer/1(Sync_In)
  Kinematics/5(lBuf) -> Forces/5(lBuf)
  Forces/8(FBuf_ext) -> Kinetics/8(FBuf_ext)
  Forces/4(Car.Load) -> Kinetics/4(Car.Load)
  Forces/7(FStabi_ext) -> Kinetics/7(FStabi_ext)
  Forces/6(FDamp_ext) -> Kinetics/6(FDamp_ext)
  Forces/5(FSpring_ext) -> Kinetics/5(FSpring_ext)
  Forces/2(Car.Virtual) -> Kinetics/2(Car.Virtual)
  Kinematics/2(lSpring) -> Forces/2(lSpring)
  Kinematics/3(vDamp) -> Forces/3(vDamp)
  Forces/3(Car.Aero) -> Kinetics/3(Car.Aero)
  Forces/1(Sync_Out) -> Kinetics/1(Sync_In)
  Kinematics/1(Sync_Out) -> Forces/1(Sync_In)
  Kinematics/4(lStabi) -> Forces/4(lStabi)

== system generic_uservehicle_truck/TruckMaker/Vehicle/IPG Vehicle/PowerTrain ==
  note: When replacing the entire powertrain,
      | be sure to disable the IPG powertrain model by using the powertrain
      | model 'Model Manager off' in the vehicle GUI.
  note: <Your model here>
  Sync_In : Inport
  Vhcl.Wheel.PT : Inport  Port=2
  VhclCtrl.PT : Inport  Port=3
  BusCreator : BusCreator  Inputs=98
  Demux : Demux  Outputs=98
      settings: DisplayOption=none
  PowerTrain : S-Function  FunctionName=TM_Sfun  Parameters='PowerTrain'  SFunctionDeploymentMode=off  EnableBusSupport=off
  PowerTrainUpd : S-Function  FunctionName=TM_Sfun  Parameters='PowerTrainUpd'  SFunctionDeploymentMode=off  EnableBusSupport=off
  Sync_Out : Outport  VectorParamsAs1DForOutWhenUnconnected=off
  wires:
  Demux/98 -> BusCreator/98  "PT IF WRR4 Trq_BrakeReg_max"
  Demux/97 -> BusCreator/97  "PT IF WRR4 Trq_BrakeReg"
  Demux/96 -> BusCreator/96  "PT IF WRR4 Trq_Supp2WC"
  Demux/95 -> BusCreator/95  "PT IF WRR4 Trq_Drive"
  Demux/94 -> BusCreator/94  "PT IF WRR4 Trq_B2W"
  Demux/93 -> BusCreator/93  "PT IF WRR4 rotv"
  Demux/92 -> BusCreator/92  "PT IF WRR4 rot"
  Demux/91 -> BusCreator/91  "PT IF WRL4 Trq_BrakeReg_max"
  Demux/90 -> BusCreator/90  "PT IF WRL4 Trq_BrakeReg"
  Demux/89 -> BusCreator/89  "PT IF WRL4 Trq_Supp2WC"
  Demux/88 -> BusCreator/88  "PT IF WRL4 Trq_Drive"
  Demux/87 -> BusCreator/87  "PT IF WRL4 Trq_B2W"
  Demux/86 -> BusCreator/86  "PT IF WRL4 rotv"
  Demux/85 -> BusCreator/85  "PT IF WRL4 rot"
  Demux/84 -> BusCreator/84  "PT IF WRR3 Trq_BrakeReg_max"
  Demux/83 -> BusCreator/83  "PT IF WRR3 Trq_BrakeReg"
  Demux/82 -> BusCreator/82  "PT IF WRR3 Trq_Supp2WC"
  Demux/81 -> BusCreator/81  "PT IF WRR3 Trq_Drive"
  Demux/80 -> BusCreator/80  "PT IF WRR3 Trq_B2W"
  Demux/79 -> BusCreator/79  "PT IF WRR3 rotv"
  Demux/78 -> BusCreator/78  "PT IF WRR3 rot"
  Demux/77 -> BusCreator/77  "PT IF WRL3 Trq_BrakeReg_max"
  Demux/76 -> BusCreator/76  "PT IF WRL3 Trq_BrakeReg"
  Demux/75 -> BusCreator/75  "PT IF WRL3 Trq_Supp2WC"
  Demux/74 -> BusCreator/74  "PT IF WRL3 Trq_Drive"
  Demux/73 -> BusCreator/73  "PT IF WRL3 Trq_B2W"
  Demux/72 -> BusCreator/72  "PT IF WRL3 rotv"
  Demux/71 -> BusCreator/71  "PT IF WRL3 rot"
  Demux/70 -> BusCreator/70  "PT IF WFR2 Trq_BrakeReg_max"
  Demux/69 -> BusCreator/69  "PT IF WFR2 Trq_BrakeReg"
  Demux/68 -> BusCreator/68  "PT IF WFR2 Trq_Supp2WC"
  Demux/67 -> BusCreator/67  "PT IF WFR2 Trq_Drive"
  Demux/66 -> BusCreator/66  "PT IF WFR2 Trq_B2W"
  Demux/65 -> BusCreator/65  "PT IF WFR2 rotv"
  Demux/64 -> BusCreator/64  "PT IF WFR2 rot"
  Demux/63 -> BusCreator/63  "PT IF WFL2 Trq_BrakeReg_max"
  Demux/62 -> BusCreator/62  "PT IF WFL2 Trq_BrakeReg"
  Demux/61 -> BusCreator/61  "PT IF WFL2 Trq_Supp2WC"
  Demux/60 -> BusCreator/60  "PT IF WFL2 Trq_Drive"
  Demux/59 -> BusCreator/59  "PT IF WFL2 Trq_B2W"
  Demux/58 -> BusCreator/58  "PT IF WFL2 rotv"
  Demux/57 -> BusCreator/57  "PT IF WFL2 rot"
  Demux/56 -> BusCreator/56  "PT IF WRR2 Trq_BrakeReg_max"
  Demux/55 -> BusCreator/55  "PT IF WRR2 Trq_BrakeReg"
  Demux/54 -> BusCreator/54  "PT IF WRR2 Trq_Supp2WC"
  Demux/53 -> BusCreator/53  "PT IF WRR2 Trq_Drive"
  Demux/52 -> BusCreator/52  "PT IF WRR2 Trq_B2W"
  Demux/51 -> BusCreator/51  "PT IF WRR2 rotv"
  Demux/50 -> BusCreator/50  "PT IF WRR2 rot"
  Demux/49 -> BusCreator/49  "PT IF WRL2 Trq_BrakeReg_max"
  Demux/48 -> BusCreator/48  "PT IF WRL2 Trq_BrakeReg"
  Demux/47 -> BusCreator/47  "PT IF WRL2 Trq_Supp2WC"
  Demux/46 -> BusCreator/46  "PT IF WRL2 Trq_Drive"
  Demux/45 -> BusCreator/45  "PT IF WRL2 Trq_B2W"
  Demux/44 -> BusCreator/44  "PT IF WRL2 rotv"
  Demux/43 -> BusCreator/43  "PT IF WRL2 rot"
  Demux/42 -> BusCreator/42  "PT IF WRR Trq_BrakeReg_max"
  Demux/41 -> BusCreator/41  "PT IF WRR Trq_BrakeReg"
  Demux/40 -> BusCreator/40  "PT IF WRR Trq_Supp2WC"
  Demux/39 -> BusCreator/39  "PT IF WRR Trq_Drive"
  Demux/38 -> BusCreator/38  "PT IF WRR Trq_B2W"
  Demux/37 -> BusCreator/37  "PT IF WRR rotv"
  Demux/36 -> BusCreator/36  "PT IF WRR rot"
  Demux/35 -> BusCreator/35  "PT IF WRL Trq_BrakeReg_max"
  Demux/34 -> BusCreator/34  "PT IF WRL Trq_BrakeReg"
  Demux/33 -> BusCreator/33  "PT IF WRL Trq_Supp2WC"
  Demux/32 -> BusCreator/32  "PT IF WRL Trq_Drive"
  Demux/31 -> BusCreator/31  "PT IF WRL Trq_B2W"
  Demux/30 -> BusCreator/30  "PT IF WRL rotv"
  Demux/29 -> BusCreator/29  "PT IF WRL rot"
  Demux/28 -> BusCreator/28  "PT IF WFR Trq_BrakeReg_max"
  Demux/27 -> BusCreator/27  "PT IF WFR Trq_BrakeReg"
  Demux/26 -> BusCreator/26  "PT IF WFR Trq_Supp2WC"
  Demux/25 -> BusCreator/25  "PT IF WFR Trq_Drive"
  Demux/24 -> BusCreator/24  "PT IF WFR Trq_B2W"
  Demux/23 -> BusCreator/23  "PT IF WFR rotv"
  Demux/22 -> BusCreator/22  "PT IF WFR rot"
  Demux/21 -> BusCreator/21  "PT IF WFL Trq_BrakeReg_max"
  Demux/20 -> BusCreator/20  "PT IF WFL Trq_BrakeReg"
  Demux/19 -> BusCreator/19  "PT IF WFL Trq_Supp2WC"
  Demux/18 -> BusCreator/18  "PT IF WFL Trq_Drive"
  Demux/17 -> BusCreator/17  "PT IF WFL Trq_B2W"
  Demux/16 -> BusCreator/16  "PT IF WFL rotv"
  Demux/15 -> BusCreator/15  "PT IF WFL rot"
  Demux/14 -> BusCreator/14  "PT IF DL_iDiff_mean"
  Demux/13 -> BusCreator/13  "PT IF Trq_Supp2BdyEng y"
  Demux/12 -> BusCreator/12  "PT IF Trq_Supp2BdyEng x"
  Demux/11 -> BusCreator/11  "PT IF Trq_Supp2Bdy1B z"
  Demux/10 -> BusCreator/10  "PT IF Trq_Supp2Bdy1B y"
  Demux/9 -> BusCreator/9  "PT IF Trq_Supp2Bdy1B x"
  Demux/8 -> BusCreator/8  "PT IF Trq_Supp2Bdy1 z"
  Demux/7 -> BusCreator/7  "PT IF Trq_Supp2Bdy1 y"
  Demux/6 -> BusCreator/6  "PT IF Trq_Supp2Bdy1 x"
  Demux/5 -> BusCreator/5  "PT IF Engine_rotv"
  Demux/4 -> BusCreator/4  "PT IF GearNo"
  Demux/3 -> BusCreator/3  "PT IF OperationError"
  Demux/2 -> BusCreator/2  "PT IF OperationState"
  Demux/1 -> BusCreator/1  "PT IF Ignition"
  BusCreator/1 -> PowerTrainUpd/2
  PowerTrain/2 -> Demux/1
  Sync_In/1 -> PowerTrain/1
  PowerTrainUpd/1 -> Sync_Out/1
  PowerTrain/1 -> PowerTrainUpd/1  "Sync"
  VhclCtrl.PT/1 -> PowerTrain/3
  Vhcl.Wheel.PT/1 -> PowerTrain/2

== system generic_uservehicle_truck/TruckMaker/Vehicle/IPG Vehicle/VehicleSource_BuiltIn ==
  u : Inport
  Compare : RelationalOperator  Operator=~=  OutDataTypeStr=boolean  ZeroCross=off  RndMeth=Nearest  InputSameDT=on
  Constant : Constant  DisableCoverage=on  Value=const  OutDataTypeStr=Inherit: Inherit via back propagation
  y : Outport  VectorParamsAs1DForOutWhenUnconnected=off
  wires:
  u/1 -> Compare/1
  Constant/1 -> Compare/2
  Compare/1 -> y/1

== system generic_uservehicle_truck/TruckMaker/Vehicle/User Vehicle (CM4SL)/Brake ==
  note: <Your model here>
  note: When replacing the entire braking system,
      | be sure to disable the IPG brake model by using the brake
      | model 'Model Manager off' in the vehicle GUI.
  Sync_In : Inport
  Brake.IF.In : Inport  Port=2
  VhclCtrl.Brake : Inport  Port=3
  Brake : S-Function  FunctionName=TM_Sfun  Parameters='Brake'  SFunctionDeploymentMode=off  EnableBusSupport=off
  BrakeUpd : S-Function  FunctionName=TM_Sfun  Parameters='BrakeUpd'  SFunctionDeploymentMode=off  EnableBusSupport=off
  BusCreator : BusCreator  Inputs=48
  CreateBus Vhcl.Wheel.PT : Subsystem
  Demux : Demux  Outputs=48
      settings: DisplayOption=none
  Sync_Out : Outport  VectorParamsAs1DForOutWhenUnconnected=off
  Vhcl.Wheel.PT : Outport  Port=2  VectorParamsAs1DForOutWhenUnconnected=off
  wires:
  Demux/1 -> BusCreator/1  "Brake IF Trq_WB FL"
  Demux/2 -> BusCreator/2  "Brake IF Trq_WB FR"
  Demux/3 -> BusCreator/3  "Brake IF Trq_WB RL"
  Demux/4 -> BusCreator/4  "Brake IF Trq_WB RR"
  Demux/5 -> BusCreator/5  "Brake IF Trq_WB RL2"
  Demux/6 -> BusCreator/6  "Brake IF Trq_WB RR2"
  Demux/7 -> BusCreator/7  "Brake IF Trq_WB FL2"
  Demux/8 -> BusCreator/8  "Brake IF Trq_WB FR2"
  Demux/9 -> BusCreator/9  "Brake IF Trq_WB RL3"
  Demux/10 -> BusCreator/10  "Brake IF Trq_WB RR3"
  Demux/11 -> BusCreator/11  "Brake IF Trq_WB RL4"
  Demux/12 -> BusCreator/12  "Brake IF Trq_WB RR4"
  Demux/13 -> BusCreator/13  "Brake IF Trq_PB FL"
  Demux/14 -> BusCreator/14  "Brake IF Trq_PB FR"
  Demux/15 -> BusCreator/15  "Brake IF Trq_PB RL"
  Demux/16 -> BusCreator/16  "Brake IF Trq_PB RR"
  Demux/17 -> BusCreator/17  "Brake IF Trq_PB RL2"
  Demux/18 -> BusCreator/18  "Brake IF Trq_PB RR2"
  Demux/19 -> BusCreator/19  "Brake IF Trq_PB FL2"
  Demux/20 -> BusCreator/20  "Brake IF Trq_PB FR2"
  Demux/21 -> BusCreator/21  "Brake IF Trq_PB RL3"
  Demux/22 -> BusCreator/22  "Brake IF Trq_PB RR3"
  Demux/23 -> BusCreator/23  "Brake IF Trq_PB RL4"
  Demux/24 -> BusCreator/24  "Brake IF Trq_PB RR4"
  Demux/25 -> BusCreator/25  "Brake IF Trq_Reg_trg FL"
  Demux/26 -> BusCreator/26  "Brake IF Trq_Reg_trg FR"
  Demux/27 -> BusCreator/27  "Brake IF Trq_Reg_trg RL"
  Demux/28 -> BusCreator/28  "Brake IF Trq_Reg_trg RR"
  Demux/29 -> BusCreator/29  "Brake IF Trq_Reg_trg RL2"
  Demux/30 -> BusCreator/30  "Brake IF Trq_Reg_trg RR2"
  Demux/31 -> BusCreator/31  "Brake IF Trq_Reg_trg FL2"
  Demux/32 -> BusCreator/32  "Brake IF Trq_Reg_trg FR2"
  Demux/33 -> BusCreator/33  "Brake IF Trq_Reg_trg RL3"
  Demux/34 -> BusCreator/34  "Brake IF Trq_Reg_trg RR3"
  Demux/35 -> BusCreator/35  "Brake IF Trq_Reg_trg RL4"
  Demux/36 -> BusCreator/36  "Brake IF Trq_Reg_trg RR4"
  Demux/37 -> BusCreator/37  "Brake IF Trq_DriveSrc_trg d0"
  Demux/38 -> BusCreator/38  "Brake IF Trq_DriveSrc_trg d1"
  Demux/39 -> BusCreator/39  "Brake IF Trq_DriveSrc_trg d2"
  Demux/40 -> BusCreator/40  "Brake IF Trq_DriveSrc_trg d3"
  Demux/41 -> BusCreator/41  "Brake IF Trq_DriveSrc_trg d4"
  Demux/42 -> BusCreator/42  "Brake IF Trq_DriveSrc_trg d5"
  Demux/43 -> BusCreator/43  "Brake IF Trq_DriveSrc_trg d6"
  Demux/44 -> BusCreator/44  "Brake IF Trq_DriveSrc_trg d7"
  Demux/45 -> BusCreator/45  "Brake IF Trq_DriveSrc_trg d8"
  Demux/46 -> BusCreator/46  "Brake IF Trq_DriveSrc_trg d9"
  Demux/47 -> BusCreator/47  "Brake IF Trq_DriveSrc_trg d10"
  Demux/48 -> BusCreator/48  "Brake IF Trq_DriveSrc_trg d11"
  BusCreator/1 -> BrakeUpd/2
  Brake/2 -> Demux/1
  BrakeUpd/1 -> Sync_Out/1
  Brake/1 -> BrakeUpd/1  "Sync"
  Brake.IF.In/1 -> Brake/2
  VhclCtrl.Brake/1 -> Brake/3
  Sync_In/1 -> Brake/1
  BrakeUpd/2 -> CreateBus Vhcl.Wheel.PT/1(In)
  CreateBus Vhcl.Wheel.PT/1(Out) -> Vhcl.Wheel.PT/1

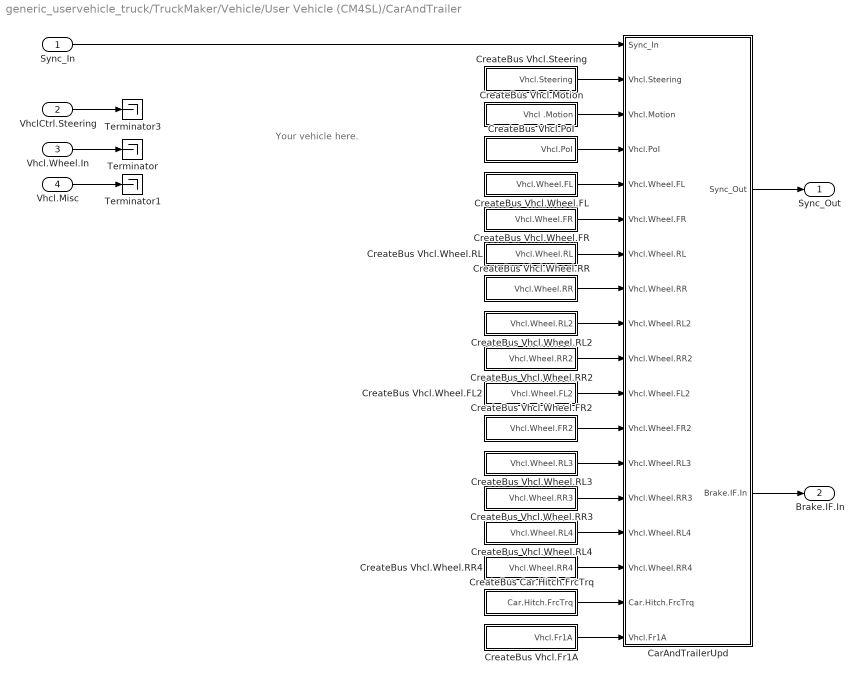
== system generic_uservehicle_truck/TruckMaker/Vehicle/User Vehicle (CM4SL)/CarAndTrailer ==
  note: Your vehicle here.
  Sync_In : Inport
  VhclCtrl.Steering : Inport  Port=2
  Vhcl.Wheel.In : Inport  Port=3
  Vhcl.Misc : Inport  Port=4
  CarAndTrailerUpd : Subsystem
  CreateBus Car.Hitch.FrcTrq : Subsystem
  CreateBus Vhcl.Fr1A : Subsystem
  CreateBus Vhcl.Motion : Subsystem
  CreateBus Vhcl.PoI : Subsystem
  CreateBus Vhcl.Steering : Subsystem
  CreateBus Vhcl.Wheel.FL : Subsystem
  CreateBus Vhcl.Wheel.FL2 : Subsystem
  CreateBus Vhcl.Wheel.FR : Subsystem
  CreateBus Vhcl.Wheel.FR2 : Subsystem
  CreateBus Vhcl.Wheel.RL : Subsystem
  CreateBus Vhcl.Wheel.RL2 : Subsystem
  CreateBus Vhcl.Wheel.RL3 : Subsystem
  CreateBus Vhcl.Wheel.RL4 : Subsystem
  CreateBus Vhcl.Wheel.RR : Subsystem
  CreateBus Vhcl.Wheel.RR2 : Subsystem
  CreateBus Vhcl.Wheel.RR3 : Subsystem
  CreateBus Vhcl.Wheel.RR4 : Subsystem
  Terminator : Terminator
  Terminator1 : Terminator
  Terminator3 : Terminator
  Sync_Out : Outport  VectorParamsAs1DForOutWhenUnconnected=off
  Brake.IF.In : Outport  Port=2  VectorParamsAs1DForOutWhenUnconnected=off
  wires:
  CreateBus Vhcl.Steering/1(Vhcl.Steering) -> CarAndTrailerUpd/2(Vhcl.Steering)
  Sync_In/1 -> CarAndTrailerUpd/1(Sync_In)
  VhclCtrl.Steering/1 -> Terminator3/1
  Vhcl.Wheel.In/1 -> Terminator/1
  Vhcl.Misc/1 -> Terminator1/1
  CarAndTrailerUpd/1(Sync_Out) -> Sync_Out/1
  CarAndTrailerUpd/2(Brake.IF.In) -> Brake.IF.In/1
  CreateBus Vhcl.Motion/1(Vhcl .Motion) -> CarAndTrailerUpd/3(Vhcl.Motion)
  CreateBus Vhcl.PoI/1(Vhcl.PoI) -> CarAndTrailerUpd/4(Vhcl.PoI)
  CreateBus Vhcl.Wheel.FL/1(Vhcl.Wheel.FL) -> CarAndTrailerUpd/5(Vhcl.Wheel.FL)
  CreateBus Vhcl.Wheel.FR/1(Vhcl.Wheel.FR) -> CarAndTrailerUpd/6(Vhcl.Wheel.FR)
  CreateBus Vhcl.Wheel.RL/1(Vhcl.Wheel.RL) -> CarAndTrailerUpd/7(Vhcl.Wheel.RL)
  CreateBus Vhcl.Wheel.RR/1(Vhcl.Wheel.RR) -> CarAndTrailerUpd/8(Vhcl.Wheel.RR)
  CreateBus Vhcl.Wheel.RL2/1(Vhcl.Wheel.RL2) -> CarAndTrailerUpd/9(Vhcl.Wheel.RL2)
  CreateBus Vhcl.Wheel.RR2/1(Vhcl.Wheel.RR2) -> CarAndTrailerUpd/10(Vhcl.Wheel.RR2)
  CreateBus Vhcl.Wheel.FL2/1(Vhcl.Wheel.FL2) -> CarAndTrailerUpd/11(Vhcl.Wheel.FL2)
  CreateBus Vhcl.Wheel.FR2/1(Vhcl.Wheel.FR2) -> CarAndTrailerUpd/12(Vhcl.Wheel.FR2)
  CreateBus Car.Hitch.FrcTrq/1(Car.Hitch.FrcTrq) -> CarAndTrailerUpd/17(Car.Hitch.FrcTrq)
  CreateBus Vhcl.Fr1A/1(Vhcl.Fr1A) -> CarAndTrailerUpd/18(Vhcl.Fr1A)
  CreateBus Vhcl.Wheel.RR3/1(Vhcl.Wheel.RR3) -> CarAndTrailerUpd/14(Vhcl.Wheel.RR3)
  CreateBus Vhcl.Wheel.RL3/1(Vhcl.Wheel.RL3) -> CarAndTrailerUpd/13(Vhcl.Wheel.RL3)
  CreateBus Vhcl.Wheel.RL4/1(Vhcl.Wheel.RL4) -> CarAndTrailerUpd/15(Vhcl.Wheel.RL4)
  CreateBus Vhcl.Wheel.RR4/1(Vhcl.Wheel.RR4) -> CarAndTrailerUpd/16(Vhcl.Wheel.RR4)
